simulink model "FPowell231"  (R2021a)
settings: Solver=VariableStepAuto  StartTime=0.0  StopTime=5  RelTol=1e-3
values from neighbouring files (symbols this model uses):
  A = [0 1 0; 0 0 1;-5 -25 -5]    [fxTransferencias.m]    (also in no-lineal-fpowel231.m = eval (A))
  B = [0; 25; -120]    [fxTransferencias.m]    (also in no-lineal-fpowel231.m = eval (B))
  C = [1 0 0]    [fxTransferencias.m]    (also in no-lineal-fpowel231.m = eval (C))
  D = [0]    [fxTransferencias.m]    (also in no-lineal-fpowel231.m = eval (D))
  i1 = 0    [no-lineal-fpowel231.m]
  u1 = 1    [no-lineal-fpowel231.m]
  v1 = 0    [no-lineal-fpowel231.m]
libraries: simulink x1
settings Model: Creator=USUARIO  LastModifiedBy=guille

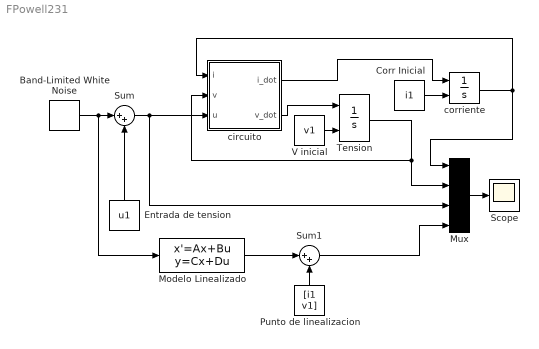
== system FPowell231 ==
  "             Entrada de tension" : Constant  Value=u1
  Band-Limited White Noise : simulink/Sources/Band-Limited White Noise  Cov=[0.00010]  Ts=0.1  seed=[23341]
  Corr Inicial : Constant  Value=i1
  Modelo Linealizado : StateSpace  A=A  B=B  C=C  D=D  InitialCondition=0
      settings: AttributesFormatString=%<Tag>
  Mux : Mux
  Punto de linealizacion : Constant  Value=[i1 v1]
  Scope : Scope
  Sum : Sum  Inputs=|++
  Sum1 : Sum  Tag=Salida Linealizada  Inputs=|++
  Tension : Integrator  InitialConditionSource=external
  V inicial : Constant  Value=v1
  circuito : MATLAB Function  TreatAsAtomicUnit=on
  corriente : Integrator  InitialConditionSource=external
  wires:
  circuito/1(i_dot) -> corriente/1
  circuito/2(v_dot) -> Tension/1
  Tension/1 -> circuito/2(v), Mux/2
  V inicial/1 -> Tension/2
  Corr Inicial/1 -> corriente/2
  "             Entrada de tension"/1 -> Sum/2
  Sum/1 -> Mux/3, circuito/3(u)
  Band-Limited White Noise/1 -> Modelo Linealizado/1, Sum/1
  Mux/1 -> Scope/1
  corriente/1 -> Mux/1, circuito/1(i)
  Modelo Linealizado/1 -> Sum1/1
  Sum1/1 -> Mux/4
  Punto de linealizacion/1 -> Sum1/2

== matlab function FPowell231/circuito ==
  data: i input; v input; u input; i_dot output; v_dot output
function [i_dot, v_dot]= circuito(i,v,u)
i_dot = -i + v;
v_dot = -i + (u-v)*(u-v-1)*(u-v-4);
